simulink model "Q13"  (R2016b)
settings: Solver=VariableStepAuto  StartTime=0.0  StopTime=20.0  RelTol=1e-3
libraries: simulink x1
settings Model: Creator=AKSHAY JP PAWAR  LastModifiedBy=AKSHAY JP PAWAR
settings DataIOCC: ReturnWorkspaceOutputs=on
settings SFSimCC: SimUseLocalCustomCode=on
settings RTWCC: RTWUseLocalCustomCode=on

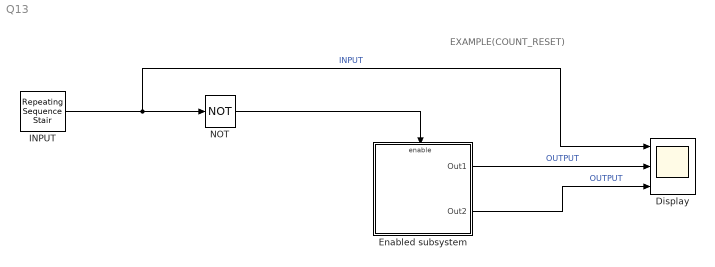
== system Q13 ==
  note: EXAMPLE(COUNT_RESET)
  Display : Scope  NumInputPorts=3
  Enabled subsystem : Subsystem
  INPUT : simulink/Sources/Repeating Sequence Stair  OutValues="[1 0  0 1 1 0 0 0 1 0 0 0 0 0 0 0 0 0 0 1 0];"  tsamp=-1  OutMin=[]  OutMax=[]  OutDataTypeStr=double  OutputDataTypeScalingMode=double  OutDataType=fixdt(0,8)  ConRadixGroup=Best Precision: Vector-wise  OutScaling=2^-12
  NOT : Logic  Operator=NOT  IconShape=distinctive  AllPortsSameDT=off  OutDataTypeStr=boolean
  wires:
  INPUT/1 -> Display/1, NOT/1  "INPUT"
  Enabled subsystem/1(Out1) -> Display/2  "OUTPUT"
  NOT/1 -> Enabled subsystem/Enable
  Enabled subsystem/2(Out2) -> Display/3  "OUTPUT"

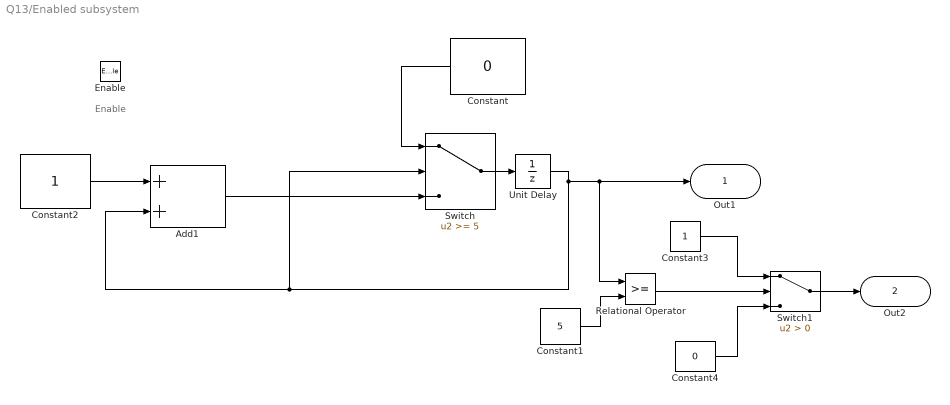
== system Q13/Enabled subsystem ==
  note: Enable
  Enable : EnablePort
  Add1 : Sum
  Constant : Constant  Value=0
  Constant1 : Constant  Value=5
  Constant2 : Constant
  Constant3 : Constant
  Constant4 : Constant  Value=0
  Relational Operator : RelationalOperator  OutDataTypeStr=boolean  RndMeth=Simplest
  Switch : Switch  Threshold=5
  Switch1 : Switch  Criteria=u2 > Threshold
  Unit Delay : UnitDelay  SampleTime=-1  HasFrameUpgradeWarning=on
  Out1 : Outport
  Out2 : Outport  Port=2
  wires:
  Constant2/1 -> Add1/1
  Add1/1 -> Switch/3
  Switch/1 -> Unit Delay/1
  Constant/1 -> Switch/1
  Unit Delay/1 -> Add1/2, Switch/2, Relational Operator/1, Out1/1
  Constant1/1 -> Relational Operator/2
  Relational Operator/1 -> Switch1/2
  Constant4/1 -> Switch1/3
  Constant3/1 -> Switch1/1
  Switch1/1 -> Out2/1
